simulink model "ansiBPF"  (R2018a)
settings: Solver=VariableStepAuto  StartTime=0.0  StopTime=0.001  RelTol=1e-3
undefined symbols (not defined in the file): fdesignblkfcn, G1, G10, G11, G12, G13, G14, G15, G16, G17, G18, G19, G2, G20, G21, G22, G23, G24, G25, G26, G3, G4, G5, G6, G7, G8, G9, gcbh, get, T
libraries: dspsrcs4 x1, dspxfrm3 x1, dspobslib x1
(part 6 of 8)

== system ansiBPF/Filter Bank /Filter 4/Bandpass Filter ==
  In : Inport
  Generated Filter Block : DiscreteFir  Tag=BlockMethodSubSystem  Coefficients=[-0.00639640017497508737 -0.000183808575014669654 -0.000185859678085867374 -0.000188700515166591629 -0.000190595492876548088 -0.000193280907967551479 -0.00019500295106286464 -0.000197542880123743701 -0.00019911206260889104 -0.000201505432291800924 -0.000202916515847706056 -0.000205182835430802515 -0.000206437516021487817 -0.000208589329099965993 -0.000209682174052230489 -0.00021172118985192555 -0.00021263828482555273 -0.000214556833858595044 -0.000215262768658975229 -0.00021703019432690594 -0.000217453456449415286 -0.000219009927256445878 -0.000219035429342216448 -0.000220292209102579596 -0.000219738660087417562 -0.000220585244791734954 -0.00021918871789526067 -0.000219576926577035123 -0.000217016605872983996 -0.000217246712974380747 -0.000213169931435971434 -0.000217400190869863099 -0.000226096874757021659 -0.000214309257912664869 -0.000216889617659619933 -0.00021435542572916075 -0.000214387726288894361 -0.000212311992474754013 -0.000211529995216927166 -0.000209473653434601897 -0.000208149606153351093 -0.000205939298847724976 -0.000204147721276272794 -0.00020171237321596388 -0.000199485640043205507 -0.000196791069795513478 -0.000194150071893684151 -0.000191187009351173018 -0.000188163675033094777 -0.000184951951678573388 -0.000181589705060233869 -0.000178165006703807308 -0.0001745049629696995 -0.000170899711295193635 -0.00016695917442367754 -0.000163168206127194354 -0.000158879814366188831 -0.000154802361132633102 -0.000149936641302610553 -0.000145375100009850224 -0.000139528528595953097 -0.00013433809409652567 -0.000127207695797959184 -0.000124037087182065161 -0.000119459472034925344 -0.000111203410456245326 -0.000106377832317852187 -9.94561897753472155e-05 -9.35710800566375369e-05 -8.66027202494845877e-05 -8.01878262905385107e-05 -7.30328459404093168e-05 -6.62018807284584101e-05 -5.87944772511833833e-05 -5.15826867461535509e-05 -4.3895416659693373e-05 -3.63091799141961519e-05 -2.83157145450075737e-05 -2.03400941452500557e-05 -1.20115420634773148e-05 -3.63331201603901982e-06 5.04228267592609493e-06 1.38167292215574411e-05 2.28206391669203916e-05 3.19508964379430592e-05 4.1221698275340067e-05 5.06247842908694672e-05 6.00761686435649726e-05 6.9683735574660986e-05 7.92949520059154283e-05 8.91885839265718367e-05 9.91012292243193611e-05 0.000109642745155544302 0.000120166217495101073 0.000131594178117420242 0.000140757864727384269 0.000151719295759991505 0.000163234555743516693 0.000173828824921519172 0.000185285516102442886 0.000196369901717889216 0.000207981932750929838 0.000219390369051235425 0.000231179685311819585 0.000242851725825094807 0.00025482557945938339 0.000266716562095736017 0.000278854115208006042 0.000290927328465638438 0.000303209504893652742 0.000315451295468035034 0.00032787864409500626 0.00034029568485542509 0.000352884182203253385 0.000365495904034018838 0.000378263406164890234 0.000391077075441364239 0.000404004875127769259 0.000416964796822729571 0.000429967183567714155 0.000442958958397996676 0.000455948364360749979 0.000468931691289575618 0.00048196741962670223 0.000495224451391110959 0.000508661841047585621 0.000522302752531917627 0.00053459832305511679 0.000548279870796822711 0.000561546011363797605 0.000574685552938410246 0.000587972325012302093 0.000601134983324684178 0.000614389182879212874 0.000627543543135088491 0.000640746458248705889 0.000653875136176830496 0.000667024930318201492 0.000680099916105053235 0.000693169652749969626 0.000706147856060866902 0.000719095649154831017 0.000731934827329682792 0.000744722327228575795 0.000757390788108903263 0.000769997268341175364 0.000782490208226856057 0.000794924233609321036 0.000807261213746303841 0.000819530183321706511 0.00083169299719354473 0.000843740026603510569 0.000855621490888570772 0.000867342424786349112 0.000878832112897290113 0.000890235436974379387 0.000901561395950063369 0.000913016544310017199 0.000924160050757658427 0.00093447787174830892 0.000945590432689845059 0.00095595142645064587 0.000966344127048270507 0.000976426389409173817 ...(+23114 chars)]  InputProcessing=Columns as channels (frame based)
  Out : Outport
  wires:
  In/1 -> Generated Filter Block/1
  Generated Filter Block/1 -> Out/1
